simulink model "washing"  (R2024b)
settings: Solver=VariableStepAuto  StartTime=0.0  StopTime=150  RelTol=1e-3
settings Model: PacingRate=4

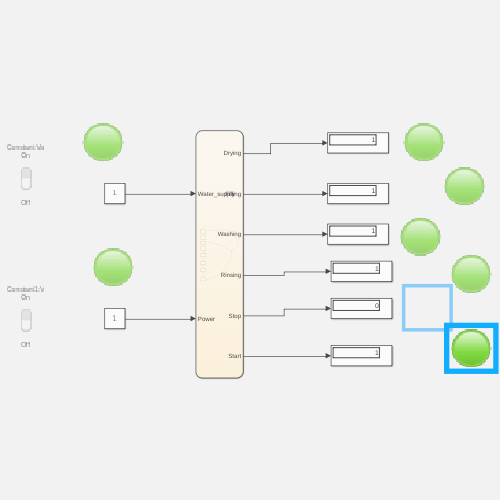
[thumbnail: Simulink's stored preview of the top-level diagram]
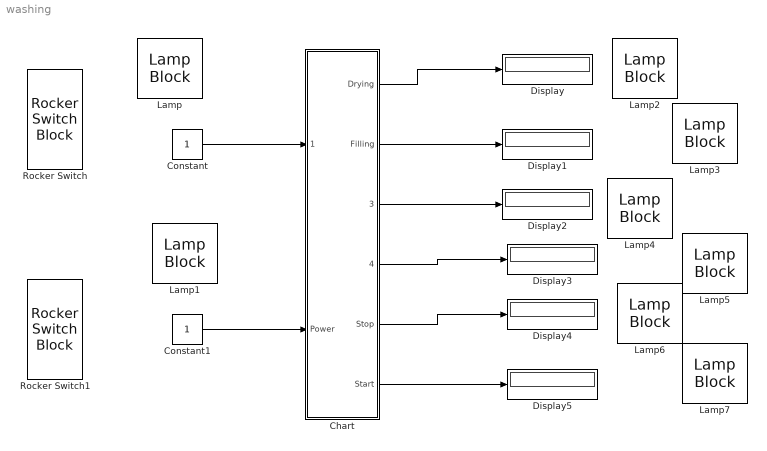
== system washing ==
  Chart : Stateflow chart  TreatAsAtomicUnit=on
  Constant : Constant
  Constant1 : Constant
  Display{,1..5} (6 alike) : Display
  Lamp{,1..7} (8 alike) : LampBlock  LabelPosition=Hide
  Rocker Switch : RockerSwitchBlock
      settings: Values={{'Off', 'On'}, [0 1]}
  Rocker Switch1 : RockerSwitchBlock
      settings: Values={{'Off', 'On'}, [0 1]}
  wires:
  Chart/1(Drying) -> Display/1
  Chart/2(Filling) -> Display1/1
  Chart/3(Washing) -> Display2/1
  Chart/4(Rinsing) -> Display3/1
  Chart/5(Stop) -> Display4/1
  Chart/6(Start) -> Display5/1
  Constant/1 -> Chart/1(Water_supply)
  Constant1/1 -> Chart/2(Power)

== stateflow chart washing/Chart ==
  state Power
  state ON
    entry:Start=1
  state Water_supply
  state Filling
    entry:Filling=1
  state Washing
    entry:Washing=1
  state Rinsing
    entry:Rinsing=1
  state Drying
    entry:Drying=1
  state OFF
    entry:Stop=1
  (default) -> Power
  Power -> (junction 17) [order 2] : [Power==0]
  Power -> ON [order 1] : [Power==1]
  (junction 17) -> (junction 18)
  ON -> Water_supply
  Water_supply -> (junction 18) [order 2] : [Water_supply==0]
  Water_supply -> Filling [order 1] : [Water_supply==1]
  Filling -> Washing : [after(50,sec)]
  (junction 18) -> OFF
  Washing -> Rinsing : [after(20,sec)]
  Rinsing -> Drying : [after(20,sec)]
  Drying -> OFF : [after(10,sec)]
  data: Water_supply input; Power input; Drying output; Filling output; Washing output; Rinsing output; Stop output; Start output
